simulink model "sldemo_hydrod"  (Simulink 7.6)
settings: Solver=ode45  SolverMode=SingleTasking  StartTime=0.0  StopTime=0.1  RelTol=1e-3  AbsTol=1e-6
model workspace (MATLAB code in the model file):
  | % Load the initial conditions and initialization data
  | % Using the same MAT file as
  | % sldemo_hydcyl.mdl
  | % sldemo_hydcyl4.mdl
  | % sldemo_hydrod.mdl
  | 
  | load sldemo_hydcyl_data;
values from neighbouring files (symbols this model uses):
  L = 67    [sldemo_foucault_data.m]
  M = (lenHouse*widHouse*htHouse+tan(pitRoof)*widHouse*lenHouse)*densAir    [sldemo_househeat_data.m]
undefined symbols (not defined in the file or in its folder): Ac, C2, I, Qmax
libraries: hydlib x4, simulink x2
Description:
  | Two Cylinder Model with Load Constraints
  | 
  | In this model, a rigid rod supporting a large mass interconnects two
  | hydraulic actuators. The model eliminates the springs as it applies the
  | piston forces directly to the load. These forces balance the
  | gravitational force and result in both linear and rotational displacement.
  | See two related demos that use the same basic components:
  | 
  | * four cylinder model: sldemo_hydcyl4.mdl
  | * single cylinder model: sldemo_hydcyl.mdl
settings Model: Creator=The MathWorks Inc.  CovMetricSettings=d  ExtModeTrigMode=oneshot  ExtModeArmWhenConnect=off  ExtModeAutoUpdateStatusClock=off
settings DataIOCC: LimitDataPoints=off  SaveFormat=Structure  SaveOutput=off  SaveState=on  SaveTime=off  SignalLoggingName=sldemo_hydrod_output
settings OptimizationCC: BlockReduction=off  BooleanDataType=off  InlineInvariantSignals=on  InitFltsAndDblsToZero=on  BufferReusableBoundary=off
settings DebuggingCC: AlgebraicLoopMsg=none  SaveWithParameterizedLinksMsg=none  SignalResolutionControl=TryResolveAllWithWarning  SolverPrmCheckMsg=none  MultiTaskDSMMsg=warning  MultiTaskCondExecSysMsg=none  SigSpecEnsureSampleTimeMsg=none  IntegerOverflowMsg=none  BusObjectLabelMismatch=none
settings HardwareCC: TargetUnknown=on
settings RTWCC: IncludeERTFirstTime=on
settings GRTTargetCC: TargetFcnLib=ansi_tfl_tmw.mat

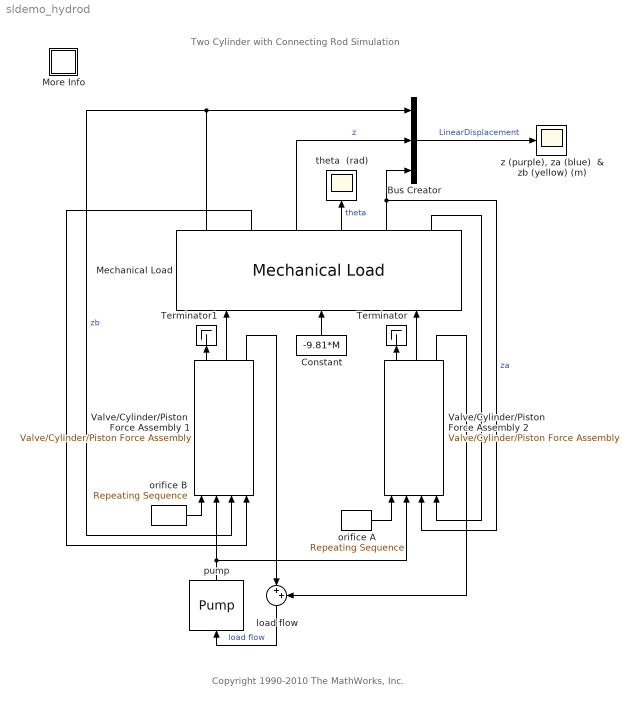
== system sldemo_hydrod ==
  note: Two Cylinder with Connecting Rod Simulation
  note: Copyright 1990-2010 The MathWorks, Inc.
  Bus Creator : BusCreator  Inputs=3
  Constant : Constant  Value=-9.81*M
  Mechanical Load : hydlib/Mechanical Load  SystemSampleTime=-1  L=L  M=M  I=I  zDotName=velocity  zName=displacement  thetaDotName=angular_velocity  thetaName=angular_displacement
  More Info : Subsystem
      settings: OpenFcn=showdemo(bdroot(gcs))
      mask Display: disp('?')
  Terminator : Terminator
  Terminator1 : Terminator
  Valve/Cylinder/Piston  Force Assembly 1 : hydlib/Valve//Cylinder//Piston Force Assembly  SystemSampleTime=-1  C1=C1  Ac=Ac  Cd=Cd  rho=rho  V30=V30  beta=Beta  p30=9.81*M/2/Ac  assemblyName=forceLeft
  Valve/Cylinder/Piston  Force Assembly 2 : hydlib/Valve//Cylinder//Piston Force Assembly  SystemSampleTime=-1  C1=C1  Ac=Ac  Cd=Cd  rho=rho  V30=V30  beta=Beta  p30=9.81*M/2/Ac  assemblyName=forceRight
  load flow : Sum  Inputs=|++  SaturateOnIntegerOverflow=on  InputSameDT=on  OutDataTypeStr=Inherit: Same as first input
  orifice A : simulink/Sources/Repeating Sequence  SystemSampleTime=-1  rep_seq_t="[0  0.1  0.2]/10"  rep_seq_y=[1 0 1]*1e-5
  orifice B : simulink/Sources/Repeating Sequence  SystemSampleTime=-1  rep_seq_t=[0 0.1 0.2]/10  rep_seq_y=[0 1 0]*1e-5
  pump : hydlib/Pump  SystemSampleTime=-1  t="[0        .04]"  Qpump=Qmax*[1 1]  p10=9.81*M/2/Ac  C2=C2/10
  theta  (rad) : Scope
      settings: TickLabels=on  TimeRange=0.1  YMin=-0.0015  YMax=0.0005  DataFormat=Array
  "z (purple), za (blue)  & zb (yellow) (m)" : Scope
      settings: TickLabels=on  TimeRange=0.1  YMin=-0.005  YMax=0.015  DataFormat=Array
  wires:
  Mechanical Load/1 -> Valve/Cylinder/Piston  Force Assembly 1/3, Bus Creator/1  "zb"
  Mechanical Load/5 -> Valve/Cylinder/Piston  Force Assembly 2/3, Bus Creator/3  "za"
  Mechanical Load/3 -> Bus Creator/2  "z"
  Mechanical Load/4 -> theta  (rad)/1  "theta"
  Constant/1 -> Mechanical Load/2
  Bus Creator/1 -> "z (purple), za (blue)  & zb (yellow) (m)"/1  "LinearDisplacement"
  Valve/Cylinder/Piston  Force Assembly 2/2 -> Mechanical Load/3
  Mechanical Load/6 -> Valve/Cylinder/Piston  Force Assembly 2/4
  orifice A/1 -> Valve/Cylinder/Piston  Force Assembly 2/1
  Valve/Cylinder/Piston  Force Assembly 2/1 -> Terminator/1
  Valve/Cylinder/Piston  Force Assembly 1/2 -> Mechanical Load/1
  Mechanical Load/2 -> Valve/Cylinder/Piston  Force Assembly 1/4
  orifice B/1 -> Valve/Cylinder/Piston  Force Assembly 1/1
  Valve/Cylinder/Piston  Force Assembly 1/1 -> Terminator1/1
  pump/1 -> Valve/Cylinder/Piston  Force Assembly 1/2, Valve/Cylinder/Piston  Force Assembly 2/2
  load flow/1 -> pump/1  "load flow"
  Valve/Cylinder/Piston  Force Assembly 2/3 -> load flow/2
  Valve/Cylinder/Piston  Force Assembly 1/3 -> load flow/1

== system sldemo_hydrod/More Info ==
